simulink model "ARDroneTT"  (R2021b)
settings: Solver=ode1  StartTime=0.0  StopTime=inf  FixedStep=sampleTime  RelTol=1e-3  EnableMultiTasking=on
values from neighbouring files (symbols this model uses):
  sampleTime = 0.065    [setupTT.m]
undefined symbols (not defined in the file or in its folder): DiscIntNeverNeededParam
libraries: ARBlocks x3, simulink x1
settings Model: SimulationMode=external  ExtModeTrigDuration=100000  Creator=Paul  LastModifiedBy=p28ma
settings SolverCC: AlgebraicLoopSolver=TrustRegion
settings DataIOCC: LimitDataPoints=on  SaveFormat=Array  SignalLoggingSaveFormat=ModelDataLogs  ReturnWorkspaceOutputs=off  TimeSaveName=time
settings OptimizationCC: ExpressionDepthLimit=2147483647  InitFltsAndDblsToZero=on
settings DebuggingCC: UnderspecifiedInitializationDetection=Classic  MergeDetectMultiDrivingBlocksExec=none  SolverPrmCheckMsg=warning  FcnCallInpInsideContextMsg=warning  StateNameClashWarn=warning  SFUnexpectedBacktrackingDiag=warning  SFNoUnconditionalDefaultTransitionDiag=warning  SFExecutionAtInitializationDiag=none  SFMachineParentedDataDiag=warning  ArithmeticOperatorsInVariantConditions=warning
settings HardwareCC: ProdBitPerLong=64  ProdHWDeviceType=Intel->x86-64 (Mac OS X)
settings ModelReferenceCC: PropagateSignalLabelsOutOfModel=off
settings SFSimCC: SimUseLocalCustomCode=off  CustomCodeUndefinedFunction=UseInterfaceOnly
settings RTWCC: Description=Simulink Desktop Real-Time  SystemTargetFile=sldrt.tlc  TemplateMakefile=sldrt.tmf  RTWUseLocalCustomCode=off  RTWCompilerOptimization=on
settings CodeAppCC: MaxIdLength=95  StateflowObjectComments=on
settings SimulinkDesktopRealTimeCC: TargetPreCompLibLocation=/Applications/MATLAB_R2017b.app/toolbox/sldrt/lib/maci64  TargetLangStandard=C89/C90 (ANSI)  SupportVariableSizeSignals=off
settings ConfigComp: CovMetricSettings=dw  CovSaveCumulativeToWorkspaceVar=on  CovSaveSingleToWorkspaceVar=on  CovExternalEMLEnable=off

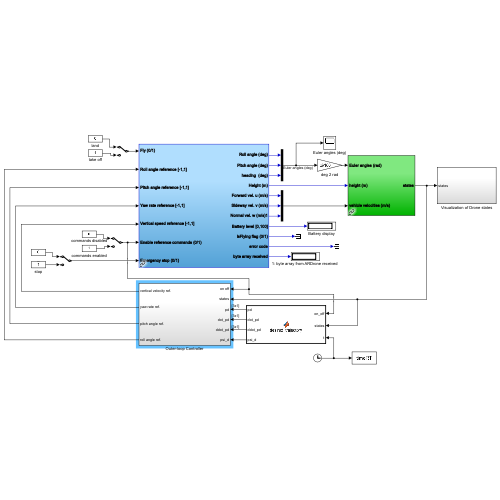
[thumbnail: Simulink's stored preview of the top-level diagram]
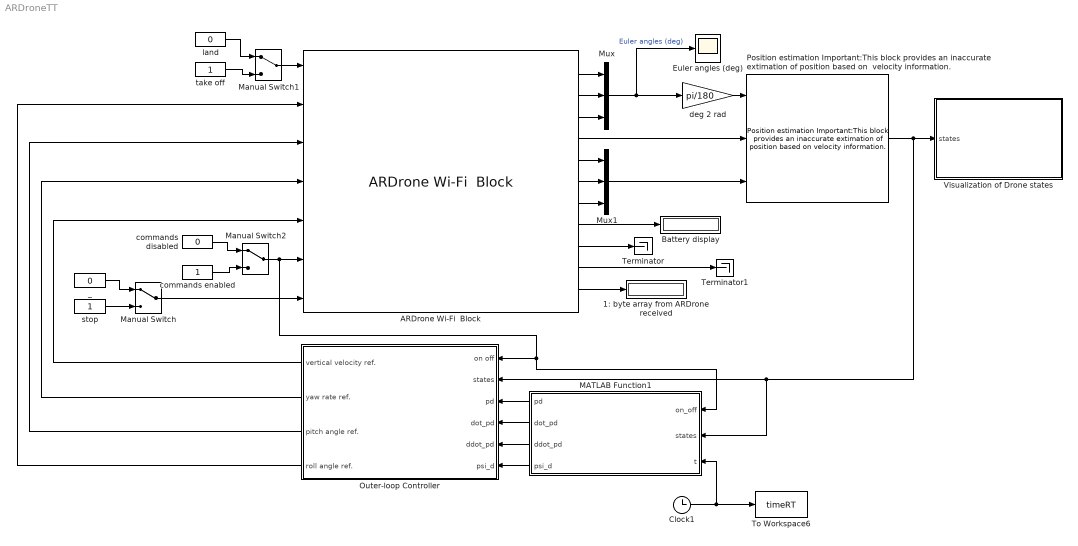
== system ARDroneTT ==
  "1: byte array from ARDrone received " : Display
  ARDrone Wi-Fi  Block : ARBlocks/ARDrone Wi-Fi  Block  SystemSampleTime=-1  VariantActivationTime=update diagram  Latency=0  AutoFrameSizeCalculation=off
  Battery display : Display
  Clock1 : Clock
  Euler angles (deg) : Scope
  MATLAB Function1 : MATLAB Function  TreatAsAtomicUnit=on  SystemSampleTime=sampleTime
  Manual Switch : ManualSwitch
  Manual Switch1 : ManualSwitch
  Manual Switch2 : ManualSwitch
  Mux : Mux  Inputs=3
  Mux1 : Mux  Inputs=3
  Outer-loop Controller : Subsystem
  "Position estimation Important:This block provides an inaccurate extimation of position based on  velocity information. " : ARBlocks/Position estimation Important:This block provides an  inaccurate extimation of position  based on  velocity information.   SystemSampleTime=-1  VariantActivationTime=update diagram  Latency=0  AutoFrameSizeCalculation=off
  Terminator : Terminator
  Terminator1 : Terminator
  To Workspace6 : ToWorkspace  VariableName=timeRT  SampleTime=sampleTime
  Visualization of Drone states : Subsystem
  _ : Constant  Value=0
  commands disabled : Constant  Value=0
  commands enabled : Constant
  deg 2 rad : Gain  Gain=pi/180
  land : Constant  Value=0
  stop : Constant
  take off : Constant
  wires:
  _/1 -> Manual Switch/1
  stop/1 -> Manual Switch/2
  land/1 -> Manual Switch1/1
  take off/1 -> Manual Switch1/2
  commands disabled/1 -> Manual Switch2/1
  commands enabled/1 -> Manual Switch2/2
  Manual Switch1/1 -> ARDrone Wi-Fi  Block/1
  Manual Switch2/1 -> MATLAB Function1/1(on_off), Outer-loop Controller/1(on off), ARDrone Wi-Fi  Block/6
  Manual Switch/1 -> ARDrone Wi-Fi  Block/7
  ARDrone Wi-Fi  Block/1 -> Mux/1
  ARDrone Wi-Fi  Block/2 -> Mux/2
  ARDrone Wi-Fi  Block/5 -> Mux1/1
  ARDrone Wi-Fi  Block/6 -> Mux1/2
  ARDrone Wi-Fi  Block/7 -> Mux1/3
  Mux/1 -> Euler angles (deg)/1, deg 2 rad/1  "Euler angles (deg)"
  ARDrone Wi-Fi  Block/8 -> Battery display/1
  Outer-loop Controller/1(vertical velocity ref.) -> ARDrone Wi-Fi  Block/5
  Outer-loop Controller/3(pitch angle ref.) -> ARDrone Wi-Fi  Block/3
  "Position estimation Important:This block provides an inaccurate extimation of position based on  velocity information. "/1 -> MATLAB Function1/2(states), Outer-loop Controller/2(states), Visualization of Drone states/1(states)
  deg 2 rad/1 -> "Position estimation Important:This block provides an inaccurate extimation of position based on  velocity information. "/1
  ARDrone Wi-Fi  Block/4 -> "Position estimation Important:This block provides an inaccurate extimation of position based on  velocity information. "/2
  Mux1/1 -> "Position estimation Important:This block provides an inaccurate extimation of position based on  velocity information. "/3
  Outer-loop Controller/4(roll angle ref.) -> ARDrone Wi-Fi  Block/2
  ARDrone Wi-Fi  Block/3 -> Mux/3
  ARDrone Wi-Fi  Block/9 -> Terminator/1
  ARDrone Wi-Fi  Block/10 -> Terminator1/1
  ARDrone Wi-Fi  Block/11 -> "1: byte array from ARDrone received "/1
  Outer-loop Controller/2(yaw rate ref.) -> ARDrone Wi-Fi  Block/4
  Clock1/1 -> MATLAB Function1/3(t), To Workspace6/1
  MATLAB Function1/1(pd) -> Outer-loop Controller/3(pd)
  MATLAB Function1/2(dot_pd) -> Outer-loop Controller/4(dot_pd)
  MATLAB Function1/3(ddot_pd) -> Outer-loop Controller/5(ddot_pd)
  MATLAB Function1/4(psi_d) -> Outer-loop Controller/6(psi_d)

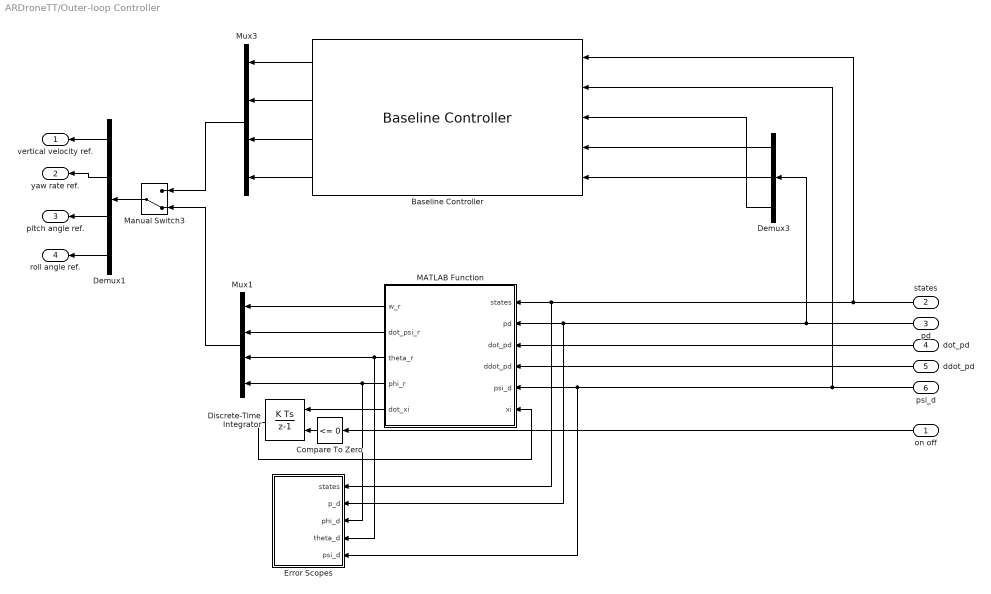
== system ARDroneTT/Outer-loop Controller ==
  on off : Inport  PortDimensions=1
  states : Inport  Port=2
  pd : Inport  Port=3  PortDimensions=[3 1]
  dot_pd : Inport  Port=4  PortDimensions=[3 1]
  ddot_pd : Inport  Port=5  PortDimensions=[3 1]
  psi_d : Inport  Port=6  PortDimensions=1
  Baseline Controller : ARBlocks/Baseline Controller  SystemSampleTime=-1  VariantActivationTime=update diagram  Latency=0  AutoFrameSizeCalculation=off
  Compare To Zero : simulink/Logic and Bit Operations/Compare To Zero  relop=<=  OutDataTypeStr=boolean
  Demux1 : Demux  Outputs=[1,1,1,1]
  Demux3 : Demux  Outputs=[1,1,1]
  Discrete-Time Integrator : DiscreteIntegrator  ExternalReset=level  InitialCondition=[0;0;0;0]  SampleTime=sampleTime  UpperSaturationLimit=10  LowerSaturationLimit=-10  ICPrevOutput=DiscIntNeverNeededParam  ICPrevScaledInput=DiscIntNeverNeededParam
  Error Scopes : Subsystem
  MATLAB Function : MATLAB Function  TreatAsAtomicUnit=on  SystemSampleTime=sampleTime
  Manual Switch3 : ManualSwitch  CurrentSetting=0
  Mux1 : Mux  Inputs=[1,1,1,1]
  Mux3 : Mux  Inputs=[1,1,1,1]
  vertical velocity ref. : Outport  VectorParamsAs1DForOutWhenUnconnected=off
  yaw rate ref. : Outport  Port=2  VectorParamsAs1DForOutWhenUnconnected=off
  pitch angle ref. : Outport  Port=3  VectorParamsAs1DForOutWhenUnconnected=off
  roll angle ref. : Outport  Port=4  VectorParamsAs1DForOutWhenUnconnected=off
  wires:
  states/1 -> Baseline Controller/1, Error Scopes/1(states), MATLAB Function/1(states)
  MATLAB Function/1(w_r) -> Mux1/1
  MATLAB Function/3(theta_r) -> Mux1/3, Error Scopes/4(theta_d)
  MATLAB Function/4(phi_r) -> Mux1/4, Error Scopes/3(phi_d)
  MATLAB Function/2(dot_psi_r) -> Mux1/2
  MATLAB Function/5(dot_xi) -> Discrete-Time Integrator/1
  Discrete-Time Integrator/1 -> MATLAB Function/6(xi)
  pd/1 -> Demux3/1, Error Scopes/2(p_d), MATLAB Function/2(pd)
  dot_pd/1 -> MATLAB Function/3(dot_pd)
  ddot_pd/1 -> MATLAB Function/4(ddot_pd)
  psi_d/1 -> Error Scopes/5(psi_d), MATLAB Function/5(psi_d), Baseline Controller/2
  Demux3/1 -> Baseline Controller/4
  Demux3/2 -> Baseline Controller/5
  Demux3/3 -> Baseline Controller/3
  Baseline Controller/4 -> Mux3/4
  Baseline Controller/3 -> Mux3/3
  Baseline Controller/2 -> Mux3/2
  Baseline Controller/1 -> Mux3/1
  Mux3/1 -> Manual Switch3/1
  Demux1/1 -> vertical velocity ref./1
  Demux1/2 -> yaw rate ref./1
  Demux1/3 -> pitch angle ref./1
  Demux1/4 -> roll angle ref./1
  Manual Switch3/1 -> Demux1/1
  Mux1/1 -> Manual Switch3/2
  on off/1 -> Compare To Zero/1
  Compare To Zero/1 -> Discrete-Time Integrator/2

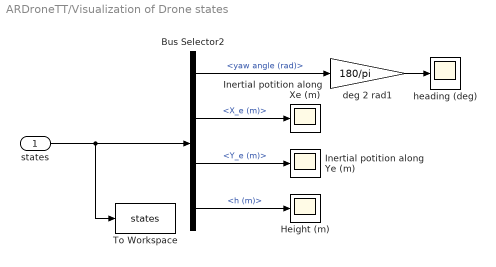
== system ARDroneTT/Visualization of Drone states ==
  states : Inport
  Bus Selector2 : BusSelector  OutputSignals=yaw angle (rad),X_e (m),Y_e (m),h (m)
  Height (m) : Scope
  Inertial potition along Xe (m) : Scope
  Inertial potition along Ye (m) : Scope
  To Workspace : ToWorkspace  VariableName=states  SaveFormat=Structure With Time  SampleTime=-1
  deg 2 rad1 : Gain  Gain=180/pi
  heading (deg) : Scope
  wires:
  states/1 -> To Workspace/1, Bus Selector2/1
  Bus Selector2/1 -> deg 2 rad1/1  "<yaw angle (rad)>"
  Bus Selector2/2 -> Inertial potition along Xe (m)/1  "<X_e (m)>"
  Bus Selector2/3 -> Inertial potition along Ye (m)/1  "<Y_e (m)>"
  Bus Selector2/4 -> Height (m)/1  "<h (m)>"
  deg 2 rad1/1 -> heading (deg)/1

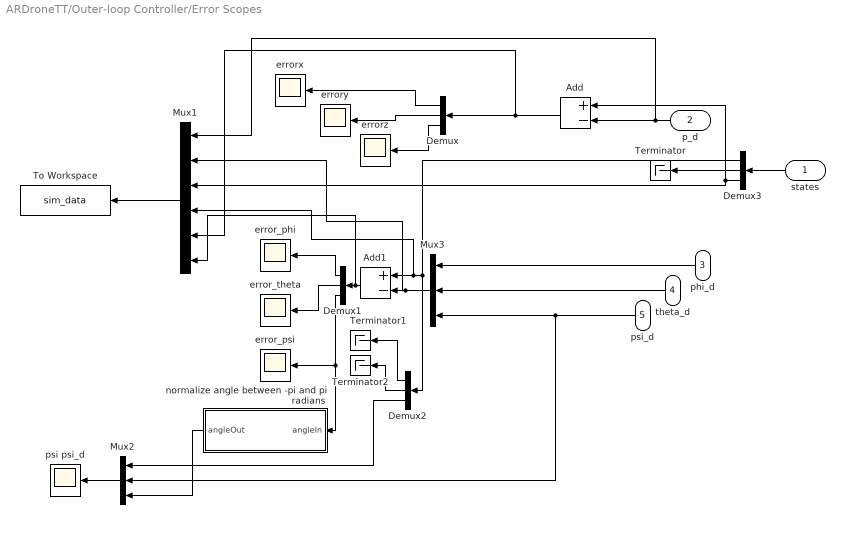
== system ARDroneTT/Outer-loop Controller/Error Scopes ==
  states : Inport
  p_d : Inport  Port=2
  phi_d : Inport  Port=3
  theta_d : Inport  Port=4
  psi_d : Inport  Port=5
  Add : Sum  Inputs=+-
  Add1 : Sum  Inputs=+-
  Demux : Demux  Outputs=3
  Demux1 : Demux  Outputs=[1,1,1]
  Demux2 : Demux  Outputs=[1,1,1]
  Demux3 : Demux  Outputs=[3,3,3]
  Mux1 : Mux  Inputs=6
  Mux2 : Mux  Inputs=[1,1,1]
  Mux3 : Mux  Inputs=[1,1,1]
  Terminator : Terminator
  Terminator1 : Terminator
  Terminator2 : Terminator
  To Workspace : ToWorkspace  VariableName=sim_data  SaveFormat=Timeseries  SampleTime=-1
  error_phi : Scope
  error_psi : Scope
  error_theta : Scope
  errorx : Scope
  errory : Scope
  errorz : Scope
  normalize angle between -pi and pi radians : MATLAB Function  TreatAsAtomicUnit=on
  psi psi_d : Scope
  wires:
  Demux/1 -> errorx/1
  Demux/3 -> errorz/1
  Demux/2 -> errory/1
  Demux1/1 -> error_phi/1
  Demux1/2 -> error_theta/1
  phi_d/1 -> Mux3/1
  theta_d/1 -> Mux3/2
  psi_d/1 -> Mux2/2, Mux3/3
  Mux2/1 -> psi psi_d/1
  Demux1/3 -> normalize angle between -pi and pi radians/1(angleIn), error_psi/1
  Demux2/3 -> Mux2/1
  normalize angle between -pi and pi radians/1(angleOut) -> Mux2/3
  states/1 -> Demux3/1
  Demux3/2 -> Terminator/1
  Demux2/1 -> Terminator1/1
  Demux2/2 -> Terminator2/1
  Add1/1 -> Mux1/6, Demux1/1
  Mux3/1 -> Mux1/2, Add1/2
  Demux3/3 -> Mux1/3, Add/1
  Demux3/1 -> Mux1/4, Add1/1, Demux2/1
  Mux1/1 -> To Workspace/1
  Add/1 -> Mux1/5, Demux/1
  p_d/1 -> Mux1/1, Add/2

== matlab function ARDroneTT/MATLAB Function1 ==
  data: on_off input; states input; t input; pd output; dot_pd output; ddot_pd output; psi_d output
function [pd, dot_pd, ddot_pd, psi_d] = desired_trajectory(on_off,states,t)
%#codegen

% ------------------------------------------------------------------------
% inputs:
% on_off - 1 if tracking is on, 0 if it is off
% states - structure with state variables
% t - current simulation time
% 
% outputs:
% pd - desired position
% dot_pd - desired velocity
% ddot_pd - desired acceleration
% psi_d - desired yaw angle
% ------------------------------------------------------------------------

persistent t0
persistent p0
persistent previous_status

on = 1;
off = 0;

if isempty(previous_status)
    previous_status = on;
    p0 = [states(7:8);-1];
end

if on_off == off
    if previous_status == on 
    % first time off or switching back off
        p0 = [states(7:8);-1]; % x0 and y0 match the current position
    end
    pd = p0;
    dot_pd = [0;0;0];
    ddot_pd = [0;0;0];
    psi_d = 0;
else
    if isempty(t0) || (previous_status == off) 
    % first time on or switching back on
        t0 = t;
        p0 = [states(7:8);-1];
    end
    dt = t-t0;

%!!!!!!!!!!!!!!!!!!!!!!!!!!!!!!!!!!!!!!!!!!!!!!!!!!!!!!!!!!!!!!!!!!!!!!!!
% replace with the necessary code to define adequate desired trajectories
% use dt, p0, and any additional parameters
    %linear
     pd = p0 + [0.3*dt;0;0];
     dot_pd = [0.3;0;0];
     ddot_pd = [0;0;0];
     psi_d = 0;

    %circle
%      pd = [cos(0.3*dt)-1;sin(0.3*dt);0];
%      dot_pd = [-0.3*sin(0.3*dt);0.3*cos(0.3*dt);0];
%      ddot_pd = [-0.09*cos(0.3*dt);-0.09*sin(0.3*dt);0];
%      %psi_d = 0;
%      psi_d = 0.3*dt;

    %3.7
%     V = 0.3;
%     delta = 1;
% 
%     pd = states(7:9);
%     pd(3) = -1;
%     psi_d = atan2(-(states(8)-0.5), delta);
%     dot_pd = [V*cos(psi_d); V*sin(psi_d); 0];
%     ddot_pd = [0;0;0];
%!!!!!!!!!!!!!!!!!!!!!!!!!!!!!!!!!!!!!!!!!!!!!!!!!!!!!!!!!!!!!!!!!!!!!!!!

end

previous_status = on_off;

== matlab function ARDroneTT/Outer-loop Controller/Error Scopes/normalize angle between -pi and pi radians ==
  data: angleIn input; angleOut output
function angleOut = fcn(angleIn)
%#codegen

angleOut = mod(angleIn, 2*pi) ;
if angleOut > pi
    angleOut = -2*pi + angleOut ; 
end

== matlab function ARDroneTT/Outer-loop Controller/MATLAB Function ==
  data: w_r output; dot_psi_r output; theta_r output; states input; pd input; dot_pd input; ddot_pd input; psi_d input; xi input; phi_r output; dot_xi output
function [w_r, dot_psi_r, theta_r, phi_r, dot_xi] = tt_controller(states, pd, dot_pd, ddot_pd,psi_d,xi)
%#codegen

% ------------------------------------------------------------------------
% inputs:
% states - structure with state variables
% pd - desired position
% dot_pd - desired velocity
% ddot_pt - desired acceleration
% psi_d - desired yaw angle
% xi - integral state (four variables)
%
% outputs:
% w_r - vertical velocity reference
% dot_psi_r - yaw rate reference
% theta_r - pitch angle reference
% phi_r - roll angle reference
% dot_xi - integral state derivative
% ------------------------------------------------------------------------

lambda = states(1:3,1); % Euler angles
psi = lambda(3);
R=euler2R(lambda);
Rz = [cos(psi) -sin(psi) 0; sin(psi) cos(psi) 0; 0 0 1];
psi_e = normalize_angle(psi-psi_d);

p = states(7:9,1); % position vector
p(3) = -p(3); % height is symmetric of z
vb = states(4:6,1); % velocity vector in body coordinates
dot_p = R*vb; % body velocity rotated to inertial frame 
dot_p(3) = -dot_p(3);

%!!!!!!!!!!!!!!!!!!!!!!!!!!!!!!!!!!!!!!!!!!!!!!!!!!!!!!!!!!!!!!!!!!!!!!
% replace with the necessary code to implement the trajectory tracking
% controller
Kp = 4;
Kd = 3;
Ki = 1;

k_w = 1;
w_r= k_w*(p(3)-pd(3));
u = -Kp*(p-pd) - Kd*(dot_p-dot_pd) - Ki*xi(1:3);
u_star = Rz'*(9.81*[0;0;1] - ddot_pd - u);

Kp_psi = 1.27767583213962;
Ki_psi = 0.316227766016838;

dot_psi_r = -Kp_psi*psi_e - Ki_psi*xi(4);
theta_r = atan2(u_star(1),u_star(3));
phi_r = atan2(-u_star(2),sqrt(u_star(1)^2+u_star(3)^2));
dot_xi = [p-pd;psi_e];
%dot_xi = [R'*(p-pd);psi_e];
%!!!!!!!!!!!!!!!!!!!!!!!!!!!!!!!!!!!!!!!!!!!!!!!!!!!!!!!!!!!!!!!!!!!!!!


function R = euler2R(l)
%#codegen
% returns the rotation matrix for a given vector of euler angles

phi = l(1); theta = l(2); psi = l(3);
R = [cos(theta)*cos(psi)...
      sin(phi)*sin(theta)*cos(psi)-cos(phi)*sin(psi)...
      cos(phi)*sin(theta)*cos(psi)+sin(phi)*sin(psi);
   cos(theta)*sin(psi)...
   sin(phi)*sin(theta)*sin(psi)+cos(phi)*cos(psi)... 
   cos(phi)*sin(theta)*sin(psi)-sin(phi)*cos(psi);
   -sin(theta)...
   sin(phi)*cos(theta)...
   cos(phi)*cos(theta)];

function angleOut = normalize_angle(angleIn)
%#codegen

angleOut = mod(angleIn, 2*pi) ;
if angleOut > pi
    angleOut = -2*pi + angleOut ; 
end
